simulink library "ENV_Library"  (R2018b)
settings: Solver=VariableStepAuto  StartTime=0.0  StopTime=10.0  RelTol=1e-3
undefined symbols (not defined in the file): c_dif, c_spe, CD, EOP, GM_EARTH, Keddy, leap, mag_data, mass, N_faces, NS, paras_dipole, R_faces, RADIUS_EARTH, RADIUS_SUN, rho_h, S_faces
libraries: MATH_library x7
settings Model: Creator=Andrea  LastModifiedBy=michele

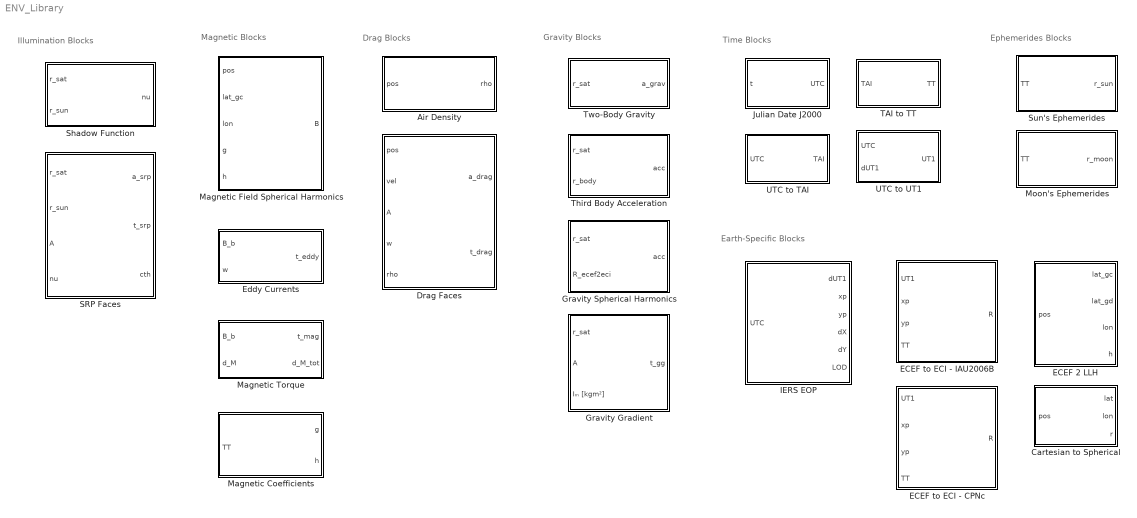
== system ENV_Library ==
  note: Illumination Blocks
  note: Magnetic Blocks
  note: Drag Blocks
  note: Gravity Blocks
  note: Earth-Specific Blocks
  note: Ephemerides Blocks
  note: Time Blocks
  Air Density : Subsystem  mask(Air Density){RBODY=RADIUS_EARTH, rho_h=rho_h}
      mask prompts: RBODY "Body Radius [m]:"; rho_h "Height-Density Look-up Table [km, kg/m³]:"
      mask help: Compute the air density at the input position, given the central body radius and a density look-up table. The input position vector must be expressed in meters.
  Cartesian to Spherical : Subsystem  mask(Cartesian to Spherical){}
      mask help: Transform a position vector in cartesian coordinates into spherical coordinates (geocentric latitude, longitude and radius)
  Drag Faces : Subsystem  mask(Drag Perturbation - Plate Model){CD=CD, m=mass, NS=NS, S_faces=S_faces, N_faces=N_faces, R_faces=R_faces}
      mask prompts: CD "Drag Coefficient [-]:"; m "Spacecraft Mass [kg]:"; NS "Number of Faces"; S_faces "Faces Areas [m²]:"; N_faces "Faces Normals:"; R_faces "Faces Centers wrt CoM [m]:"
      mask help: Compute the drag acceleration and torque by modelling the spacecraft as a collection of plates. It is valid only for the Earth (because it exploits its angular velocity). All the input vectors must be expressed in the Inertial Frame in [m] and [m/s]
      mask DialogControl ParameterGroupVar Prompt: Spacecraft Properties
      mask DialogControl Container3 Prompt: Spacecraft Geometry
  "ECEF 2 LLH  " : Subsystem  mask(ECEF to LLH){}
      mask help: Transform a position vector in ECEF coordinates to geodetic latitude, longitude and altitude from the reference WGS84 ellipsoid. The input vector and output height are expressed in meters.
  ECEF to ECI - CPNc : Subsystem  mask(ECEF to ECI	 - CPNc){}
      mask help:
      | Compute the Position Rotation Matrix from the ECEF to the ECI reference frame using the IERS 2010 Conventions (CPNc approximate Capitaine model) and the Earth Orientation Parameters.
      |
      | The CPNc version is a concise model with a cut-off at 2.5 mas of the X and Y series, delivering a worst-case accuracy of about 15 mas between 1995-2050. It does not take into account the Free Core Nutation (~0.2 mas)
  ECEF to ECI - IAU2006B : Subsystem  mask(ECEF to ECI){}
      mask help: Compute the Position Rotation Matrix from the ECEF to the ECI reference frame using the IERS 2010 Conventions (IAU2006/2000B precession-nutation model) and the Earth Orientation Parameters.
  Eddy Currents : Subsystem  mask(Eddy Currents Torque){Ke=Keddy}
      mask prompts: Ke "Eddy current coefficient:"
      mask help: Compute the magnetic torque induced by Eddy currents in [Nm].
  Gravity Gradient : Subsystem  mask(Gravity Gradient Torque){GM=GM_EARTH}
      mask prompts: GM "Gravitational planetary constant:"
      mask help: Compute the gravity gradient torque in [Nm], given the satellite position, the DCM from the inertial to body frame and the spacecraft inertia matrix. The position vector and the planetary gravitational constant must be expressed in the same units (i.e., m and m³/s²).
  Gravity Spherical Harmonics : Subsystem  mask{GRAV=0}
      mask prompts: GRAV "Spherical Gravity Model Structure:"
      mask DialogControl DescGroupVar Prompt: Gravity Spherical Harmonics
      mask DialogControl DescTextVar Prompt: Compute the perturbing gravitational acceleration using a spherical harmonic expansions. The input position and output acceleration vectors are expressed in the inertial reference frame.
  IERS EOP : Subsystem  mask(Earth Orientation Parameters){EOP=EOP}
      mask prompts: EOP "EOP Data Structure:"
      mask help: Interpolate the IERS EOP data at the given input UTC seconds since J2000.
      mask DialogControl Container2 Prompt: Parameters
  Julian Date J2000 : Subsystem  mask(Julian Date){jd0=0}
      mask prompts: jd0 "Start Julian Date [days]"
      mask help: Return the current simulation time in UTC seconds since J2000. The input time t expresses the seconds elapsed since the starting Julian Date jd0.
  Magnetic Coefficients : Subsystem  mask(Magnetic Field Coefficients){mag_data=0}
      mask prompts: mag_data "Magnetic Field Data:"
      mask help: Compute the magnetic field expansion coefficients at epoch using IGRF's coefficients and their secular variation.
  "Magnetic Field Spherical Harmonics  " : Subsystem  mask(Magnetic Field Vector){mag_data=mag_data}
      mask prompts: mag_data "Magnetic Field Data:"
      mask help: Compute the magnetic field vector in the Inertial frame using the spherical harmonic expansion and IGRF13's coefficients (at epoch). The inputs must be in [m] and [rad].
  Magnetic Torque : Subsystem  mask(Magnetic Torque){parasitic=paras_dipole}
      mask prompts: parasitic "Parasitic Magnetic Dipole [Am²]:"
      mask help: Compute the magnetic perturbing torque in [Nm] given the magnetic field vector in the body frame and the magnetic control dipole.
  Moon's Ephemerides : Subsystem  mask(Moon's Ephemerides){}
      mask help: Compute the Moon's position using low-precision ephemerides. The output position vector is expressed in a True-of-Date geocentric frame in [km].
  "SRP Faces " : Subsystem  mask(SRP Perturbation - Plate Model){m=mass, c_dif=c_dif, c_spe=c_spe, NS=NS, S_faces=S_faces, N_faces=N_faces, R_faces=R_faces}
      mask prompts: m "Spacecraft Mass [kg]:"; c_dif "Diffuse Coefficient [-]:"; c_spe "Specular Coefficient [-]:"; NS "Number of Faces"; S_faces "Faces Areas [m²]:"; N_faces "Faces Normals:"; R_faces "Faces Center of Pressures wrt CoM [m]:"
      mask help: Compute the Solar Radiation Pressure (SRP) acceleration and torque by modelling the spacecraft as a collection of plates. All the input vectors must be in [m]. The shadow function nu is used to trigger the perturbations.
      mask DialogControl ParameterGroupVar Prompt: Spacecraft Properties
      mask DialogControl Container3 Prompt: Optical Properties
      mask DialogControl Container4 Prompt: Spacecraft Geometry
  "Shadow Function " : Subsystem  mask(Shadow Function){Rsun=RADIUS_SUN, Rbody=RADIUS_EARTH}
      mask prompts: Rsun "Radius of the Sun:"; Rbody "Radius of the Occulting Body"
      mask help: Compute the dimensionless shadow function coefficient (i.e., the luminosity ratio). All the inputs must be expressed in the same units.
  Sun's Ephemerides : Subsystem  mask(Sun's Ephemerides){}
      mask help: Compute the Sun's position using low-precision ephemerides. The output position vector is expressed in a True-of-Date geocentric frame in [km].
  TAI to TT : Subsystem  mask(TAI to TT){}
      mask help: Convert seconds since J2000 from the International Atomic Time (TAI) to the Terrestrial Time (TT) scale.
  Third Body Acceleration : Subsystem  mask(Third-Body Perturbation){GM=-3}
      mask prompts: GM "Third: Body Gravitational Constant"
      mask help: Compute the third-body gravitational perturbation, given the spacecraft and the third-body positions with respect to the central body. The input vectors and the planetary gravitational constant must be expressed in the same units of length (i.e., m and m³/s²).
  Two-Body Gravity : Subsystem  mask(Two-Body Acceleration){GM=0}
      mask prompts: GM "Planetary Gravitational Constant:"
      mask help: Compute the gravitational acceleration using the Two-Body Keplerian model. The input vector and the gravitational constant must have the same units of length (i.e., m and m³/s²).
  UTC to TAI : Subsystem  mask(UTC to TAI){leapseconds=leap}
      mask prompts: leapseconds "Leapseconds [s]:"
      mask help: Convert UTC seconds since J2000 to seconds in the International Atomic Time (TAI) scale. This block assumes that no leapseconds are added throughout the simulation.
      mask DialogControl Container2 Prompt: Parameters
  UTC to UT1 : Subsystem  mask(UTC to UT1){}
      mask help: Convert seconds since J2000 from the UTC to the UT1 scale. The additional dUT1 input must also be expressed in seconds.

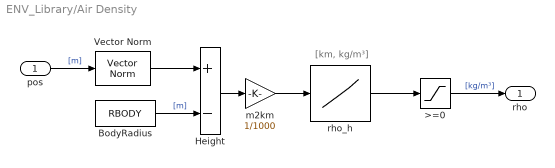
== system ENV_Library/Air Density ==
  note: [km, kg/m³]
  pos : Inport
  >=0 : Saturate  UpperLimit=Inf  LowerLimit=0
  BodyRadius : Constant  Value=RBODY
  Height : Sum  Inputs=+-
  Vector Norm : MATH_library/Vector Norm
  m2km : Gain  Gain=1/1000
  rho_h : Lookup_n-D  NumberOfTableDimensions=1  BreakpointsForDimension1=rho_h(:,1)  Table=rho_h(:,2)  DiagnosticForOutOfRangeInput=Warning  InternalRulePriority=Speed  RndMeth=Simplest  InputSameDT=on
  "rho " : Outport
  wires:
  >=0/1 -> "rho "/1  "[kg/m³]"
  pos/1 -> Vector Norm/1  "[m]"
  rho_h/1 -> >=0/1
  Height/1 -> m2km/1
  BodyRadius/1 -> Height/2  "[m]"
  Vector Norm/1 -> Height/1
  m2km/1 -> rho_h/1

== system ENV_Library/Cartesian to Spherical ==
  note: [m]
  note: [rad]
  note: [m]
  note: [rad]
  pos : Inport
  MATLAB Function : MATLAB Function  TreatAsAtomicUnit=on
  lat : Outport
  lon : Outport  Port=2
  " r" : Outport  Port=3
  wires:
  MATLAB Function/3(r) -> " r"/1
  MATLAB Function/2(lon) -> lon/1
  MATLAB Function/1(lat) -> lat/1
  pos/1 -> MATLAB Function/1(pos)

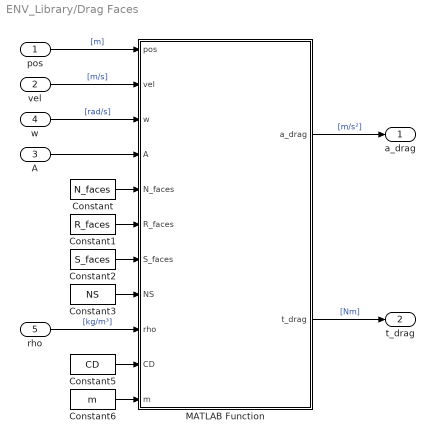
== system ENV_Library/Drag Faces ==
  pos : Inport
  vel : Inport  Port=2
  A : Inport  Port=3
  w : Inport  Port=4
  rho : Inport  Port=5
  Constant : Constant  Value=N_faces
  Constant1 : Constant  Value=R_faces
  Constant2 : Constant  Value=S_faces
  Constant3 : Constant  Value=NS
  Constant5 : Constant  Value=CD
  Constant6 : Constant  Value=m
  MATLAB Function : MATLAB Function  TreatAsAtomicUnit=on
  a_drag : Outport
  t_drag : Outport  Port=2
  wires:
  w/1 -> MATLAB Function/3(w)  "[rad/s]"
  MATLAB Function/2(t_drag) -> t_drag/1  "[Nm]"
  Constant6/1 -> MATLAB Function/11(m)
  Constant5/1 -> MATLAB Function/10(CD)
  rho/1 -> MATLAB Function/9(rho)  "[kg/m³]"
  Constant3/1 -> MATLAB Function/8(NS)
  Constant2/1 -> MATLAB Function/7(S_faces)
  Constant1/1 -> MATLAB Function/6(R_faces)
  Constant/1 -> MATLAB Function/5(N_faces)
  A/1 -> MATLAB Function/4(A)
  MATLAB Function/1(a_drag) -> a_drag/1  "[m/s²]"
  vel/1 -> MATLAB Function/2(vel)  "[m/s]"
  pos/1 -> MATLAB Function/1(pos)  "[m]"

== system ENV_Library/ECEF 2 LLH   ==
  note: [rad]
  note: [m]
  note: [rad]
  note: [m]
  note: [rad]
  pos : Inport
  MATLAB Function : MATLAB Function  TreatAsAtomicUnit=on
  lat_gc : Outport
  lat_gd : Outport  Port=2
  lon : Outport  Port=3
  " h" : Outport  Port=4
  wires:
  MATLAB Function/4(h) -> " h"/1
  MATLAB Function/3(lon) -> lon/1
  MATLAB Function/1(lat_gc) -> lat_gc/1
  pos/1 -> MATLAB Function/1(pos)
  MATLAB Function/2(lat_gd) -> lat_gd/1

== system ENV_Library/ECEF to ECI - CPNc ==
  note: [sec]
  note: [sec]
  note: [rad]
  note: [rad]
  UT1 : Inport
  xp : Inport  Port=2
  yp : Inport  Port=3
  TT : Inport  Port=4
  MATLAB Function : MATLAB Function  TreatAsAtomicUnit=on
  R : Outport
  wires:
  UT1/1 -> MATLAB Function/2(ut1_s)
  MATLAB Function/1(R) -> R/1
  TT/1 -> MATLAB Function/1(tt_s)
  xp/1 -> MATLAB Function/3(xp)
  yp/1 -> MATLAB Function/4(yp)

== system ENV_Library/ECEF to ECI - IAU2006B ==
  UT1 : Inport
  xp : Inport  Port=2
  yp : Inport  Port=3
  TT : Inport  Port=4
  MATLAB Function : MATLAB Function  TreatAsAtomicUnit=on
  R : Outport
  wires:
  yp/1 -> MATLAB Function/4(yp)  "[rad]"
  xp/1 -> MATLAB Function/3(xp)  "[rad]"
  UT1/1 -> MATLAB Function/2(ut1_s)  "[sec]"
  MATLAB Function/1(R) -> R/1
  TT/1 -> MATLAB Function/1(tt_s)  "[sec]"

== system ENV_Library/Eddy Currents ==
  B_b : Inport
  w : Inport  Port=2
  Cross Product : MATH_library/Cross Product
  Cross Product1 : MATH_library/Cross Product
  Gain : Gain  Gain=Ke
  t_eddy : Outport
  wires:
  Gain/1 -> t_eddy/1  "[Nm]"
  Cross Product1/1 -> Gain/1
  B_b/1 -> Cross Product1/2, Cross Product/2  "[T]"
  Cross Product/1 -> Cross Product1/1
  w/1 -> Cross Product/1  "[rad]"

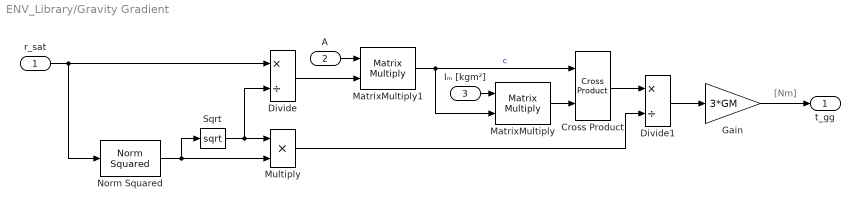
== system ENV_Library/Gravity Gradient ==
  note: [Nm]
  r_sat : Inport
  A : Inport  Port=2
  Iₘ [kgm²] : Inport  Port=3
  Cross Product : MATH_library/Cross Product
  Divide : Product  Inputs=*/
  Divide1 : Product  Inputs=*/
  Gain : Gain  Gain=3*GM
  MatrixMultiply : Product  Multiplication=Matrix(*)
  MatrixMultiply1 : Product  Multiplication=Matrix(*)
  Multiply : Product
  Norm Squared : MATH_library/Norm Squared
  Sqrt : Sqrt  SaturateOnIntegerOverflow=on
  t_gg : Outport
  wires:
  Gain/1 -> t_gg/1
  r_sat/1 -> Norm Squared/1, Divide/1
  Iₘ [kgm²]/1 -> MatrixMultiply/1
  Norm Squared/1 -> Sqrt/1, Multiply/2
  Sqrt/1 -> Divide/2, Multiply/1
  A/1 -> MatrixMultiply1/1
  Divide/1 -> MatrixMultiply1/2
  MatrixMultiply1/1 -> Cross Product/1, MatrixMultiply/2  "c"
  MatrixMultiply/1 -> Cross Product/2
  Cross Product/1 -> Divide1/1
  Multiply/1 -> Divide1/2
  Divide1/1 -> Gain/1

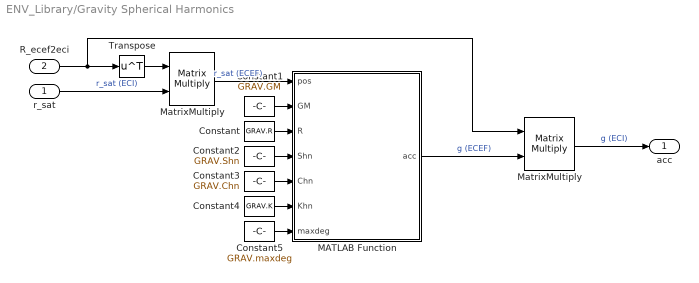
== system ENV_Library/Gravity Spherical Harmonics ==
  r_sat : Inport
  R_ecef2eci : Inport  Port=2
  Constant : Constant  Value=GRAV.R
  Constant1 : Constant  Value=GRAV.GM
  Constant2 : Constant  Value=GRAV.Shn
  Constant3 : Constant  Value=GRAV.Chn
  Constant4 : Constant  Value=GRAV.K
  Constant5 : Constant  Value=GRAV.maxdeg
  MATLAB Function : MATLAB Function  TreatAsAtomicUnit=on
  MatrixMultiply : Product  Multiplication=Matrix(*)
  "MatrixMultiply   " : Product  Multiplication=Matrix(*)
  Transpose : Math  Operator=transpose  SaturateOnIntegerOverflow=on
  acc : Outport
  wires:
  Constant/1 -> MATLAB Function/3(R)
  Constant1/1 -> MATLAB Function/2(GM)
  Constant2/1 -> MATLAB Function/4(Shn)
  Constant3/1 -> MATLAB Function/5(Chn)
  Constant4/1 -> MATLAB Function/6(Khn)
  Constant5/1 -> MATLAB Function/7(maxdeg)
  MatrixMultiply/1 -> acc/1  "g (ECI)"
  MATLAB Function/1(acc) -> MatrixMultiply/2  "g (ECEF)"
  R_ecef2eci/1 -> MatrixMultiply/1, Transpose/1
  "MatrixMultiply   "/1 -> MATLAB Function/1(pos)  "r_sat (ECEF)"
  r_sat/1 -> "MatrixMultiply   "/2  "r_sat (ECI)"
  Transpose/1 -> "MatrixMultiply   "/1

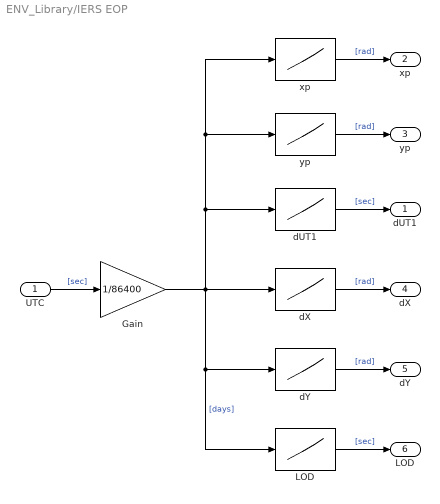
== system ENV_Library/IERS EOP ==
  UTC : Inport
  Gain : Gain  Gain=1/86400
  LOD : Lookup_n-D  NumberOfTableDimensions=1  BreakpointsForDimension1=EOP.jd  Table=EOP.LOD  DiagnosticForOutOfRangeInput=Warning  InternalRulePriority=Speed  RndMeth=Simplest  InputSameDT=on
  dUT1 : Lookup_n-D  NumberOfTableDimensions=1  BreakpointsForDimension1=EOP.jd  Table=EOP.dut1  DiagnosticForOutOfRangeInput=Warning  InternalRulePriority=Speed  RndMeth=Simplest  InputSameDT=on
  dX : Lookup_n-D  NumberOfTableDimensions=1  BreakpointsForDimension1=EOP.jd  Table=EOP.dx  DiagnosticForOutOfRangeInput=Warning  InternalRulePriority=Speed  RndMeth=Simplest  InputSameDT=on
  dY : Lookup_n-D  NumberOfTableDimensions=1  BreakpointsForDimension1=EOP.jd  Table=EOP.dy  DiagnosticForOutOfRangeInput=Warning  InternalRulePriority=Speed  RndMeth=Simplest  InputSameDT=on
  xp : Lookup_n-D  NumberOfTableDimensions=1  BreakpointsForDimension1=EOP.jd  Table=EOP.xp  DiagnosticForOutOfRangeInput=Warning  InternalRulePriority=Speed  RndMeth=Simplest  InputSameDT=on
  yp : Lookup_n-D  NumberOfTableDimensions=1  BreakpointsForDimension1=EOP.jd  Table=EOP.yp  DiagnosticForOutOfRangeInput=Warning  InternalRulePriority=Speed  RndMeth=Simplest  InputSameDT=on
  " dUT1" : Outport
  " xp" : Outport  Port=2
  " yp" : Outport  Port=3
  " dX" : Outport  Port=4
  " dY" : Outport  Port=5
  " LOD" : Outport  Port=6
  wires:
  Gain/1 -> LOD/1, dY/1, dX/1, dUT1/1, yp/1, xp/1  "[days]"
  dY/1 -> " dY"/1  "[rad]"
  LOD/1 -> " LOD"/1  "[sec]"
  dX/1 -> " dX"/1  "[rad]"
  xp/1 -> " xp"/1  "[rad]"
  yp/1 -> " yp"/1  "[rad]"
  UTC/1 -> Gain/1  "[sec]"
  dUT1/1 -> " dUT1"/1  "[sec]"

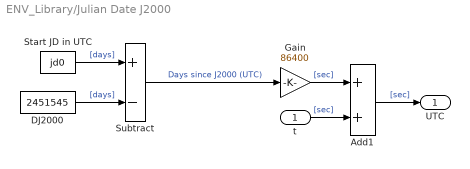
== system ENV_Library/Julian Date J2000 ==
  t : Inport
  Add1 : Sum
  DJ2000 : Constant  Value=2451545
  Gain : Gain  Gain=86400
  "Start JD in UTC " : Constant  Value=jd0
  Subtract : Sum  Inputs=+-
  UTC : Outport
  wires:
  Gain/1 -> Add1/1  "[sec]"
  Subtract/1 -> Gain/1  "Days since J2000 (UTC)"
  DJ2000/1 -> Subtract/2  "[days]"
  "Start JD in UTC "/1 -> Subtract/1  "[days]"
  Add1/1 -> UTC/1  "[sec]"
  t/1 -> Add1/2  "[sec]"

== system ENV_Library/Magnetic Coefficients ==
  note: [sec]
  TT : Inport
  Constant : Constant  Value=mag_data
  MATLAB Function : MATLAB Function  TreatAsAtomicUnit=on
  g : Outport
  h : Outport  Port=2
  wires:
  TT/1 -> MATLAB Function/1(time)
  MATLAB Function/1(g) -> g/1
  MATLAB Function/2(h) -> h/1
  Constant/1 -> MATLAB Function/2(data)

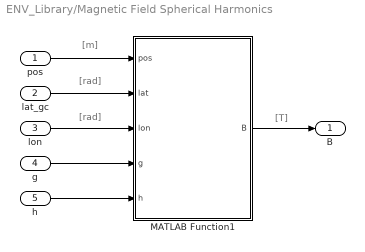
== system ENV_Library/Magnetic Field Spherical Harmonics   ==
  note: [m]
  note: [rad]
  note: [rad]
  note: [T]
  pos : Inport
  lat_gc : Inport  Port=2
  lon : Inport  Port=3
  g : Inport  Port=4
  h : Inport  Port=5
  MATLAB Function1 : MATLAB Function  TreatAsAtomicUnit=on
  B : Outport
  wires:
  g/1 -> MATLAB Function1/4(g)
  pos/1 -> MATLAB Function1/1(pos)
  lon/1 -> MATLAB Function1/3(lon)
  lat_gc/1 -> MATLAB Function1/2(lat)
  MATLAB Function1/1(B) -> B/1
  h/1 -> MATLAB Function1/5(h)

== system ENV_Library/Magnetic Torque ==
  note: [T]
  note: [Am²]
  note: [Nm]
  note: [Am²]
  B_b : Inport
  d_M : Inport  Port=2
  Constant : Constant  Value=parasitic
  Cross Product : MATH_library/Cross Product
  Subtract : Sum
  t_mag : Outport
  d_M_tot : Outport  Port=2
  wires:
  Cross Product/1 -> t_mag/1
  Subtract/1 -> Cross Product/1, d_M_tot/1
  Constant/1 -> Subtract/2
  d_M/1 -> Subtract/1
  B_b/1 -> Cross Product/2

== system ENV_Library/Moon's Ephemerides ==
  TT : Inport
  MoonEphemeris : MATLAB Function  TreatAsAtomicUnit=on
  r_moon : Outport
  wires:
  MoonEphemeris/1(pos) -> r_moon/1
  TT/1 -> MoonEphemeris/1(time)  "[sec]"

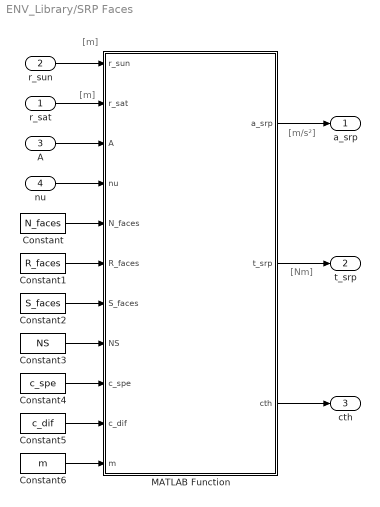
== system ENV_Library/SRP Faces  ==
  note: [m]
  note: [m]
  note: [Nm]
  note: [m/s²]
  r_sat : Inport
  r_sun : Inport  Port=2
  A : Inport  Port=3
  nu : Inport  Port=4
  Constant : Constant  Value=N_faces
  Constant1 : Constant  Value=R_faces
  Constant2 : Constant  Value=S_faces
  Constant3 : Constant  Value=NS
  Constant4 : Constant  Value=c_spe
  Constant5 : Constant  Value=c_dif
  Constant6 : Constant  Value=m
  MATLAB Function : MATLAB Function  TreatAsAtomicUnit=on
  a_srp : Outport
  t_srp : Outport  Port=2
  cth : Outport  Port=3
  wires:
  MATLAB Function/3(cth) -> cth/1
  MATLAB Function/2(t_srp) -> t_srp/1
  Constant6/1 -> MATLAB Function/11(m)
  Constant5/1 -> MATLAB Function/10(c_dif)
  Constant4/1 -> MATLAB Function/9(c_spe)
  Constant3/1 -> MATLAB Function/8(NS)
  Constant2/1 -> MATLAB Function/7(S_faces)
  Constant1/1 -> MATLAB Function/6(R_faces)
  Constant/1 -> MATLAB Function/5(N_faces)
  nu/1 -> MATLAB Function/4(nu)
  A/1 -> MATLAB Function/3(A)
  r_sun/1 -> MATLAB Function/1(r_sun)
  r_sat/1 -> MATLAB Function/2(r_sat)
  MATLAB Function/1(a_srp) -> a_srp/1

== system ENV_Library/Shadow Function  ==
  note: [m]
  note: [m]
  r_sat : Inport
  r_sun : Inport  Port=2
  Constant : Constant  Value=Rsun
  Constant1 : Constant  Value=Rbody
  MATLAB Function : MATLAB Function  TreatAsAtomicUnit=on
  nu : Outport
  wires:
  Constant1/1 -> MATLAB Function/4(Rp)
  Constant/1 -> MATLAB Function/3(Rs)
  r_sun/1 -> MATLAB Function/2(r_sun)
  r_sat/1 -> MATLAB Function/1(r_sat)
  MATLAB Function/1(nu) -> nu/1

== system ENV_Library/Sun's Ephemerides ==
  TT : Inport
  SunEphemeris : MATLAB Function  TreatAsAtomicUnit=on
  r_sun : Outport
  wires:
  SunEphemeris/1(pos) -> r_sun/1
  TT/1 -> SunEphemeris/1(time)  "[sec]"

== system ENV_Library/TAI to TT ==
  TAI : Inport
  Add1 : Sum
  Constant : Constant  Value=32.184
  TT : Outport
  wires:
  Constant/1 -> Add1/1  "[sec]"
  Add1/1 -> TT/1  "[sec]"
  TAI/1 -> Add1/2  "[sec]"

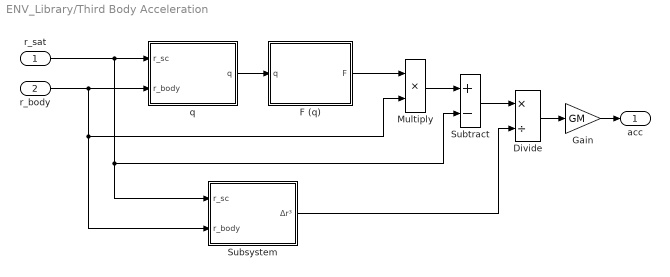
== system ENV_Library/Third Body Acceleration ==
  r_sat : Inport
  r_body : Inport  Port=2
  Divide : Product  Inputs=*/
  F (q) : Subsystem
  Gain : Gain  Gain=GM
  Multiply : Product
  Subsystem : Subsystem
  Subtract : Sum  Inputs=+-
  q : Subsystem
  acc : Outport
  wires:
  r_sat/1 -> Subsystem/1(r_sc), Subtract/2, q/1(r_sc)
  q/1(q) -> F (q)/1(q)
  r_body/1 -> Subsystem/2(r_body), Multiply/2, q/2(r_body)
  F (q)/1(F) -> Multiply/1
  Multiply/1 -> Subtract/1
  Subtract/1 -> Divide/1
  Subsystem/1(Δr³) -> Divide/2
  Divide/1 -> Gain/1
  Gain/1 -> acc/1

== system ENV_Library/Two-Body Gravity ==
  r_sat : Inport
  Divide : Product  Inputs=*/
  Gain : Gain  Gain=-GM
  Multiply : Product
  Norm Squared : MATH_library/Norm Squared
  Sqrt : Sqrt  SaturateOnIntegerOverflow=on
  a_grav : Outport
  wires:
  Gain/1 -> a_grav/1
  Norm Squared/1 -> Multiply/1, Sqrt/1
  r_sat/1 -> Norm Squared/1, Divide/1
  Divide/1 -> Gain/1
  Sqrt/1 -> Multiply/2
  Multiply/1 -> Divide/2

== system ENV_Library/UTC to TAI ==
  UTC : Inport
  Constant : Constant  Value=leapseconds
  Subtract : Sum
  TAI : Outport
  wires:
  Subtract/1 -> TAI/1  "[sec]"
  UTC/1 -> Subtract/2  "[sec]"
  Constant/1 -> Subtract/1  "[sec]"

== system ENV_Library/UTC to UT1 ==
  UTC : Inport
  dUT1 : Inport  Port=2
  Add1 : Sum
  UT1 : Outport
  wires:
  dUT1/1 -> Add1/1  "[sec]"
  Add1/1 -> UT1/1  "[sec]"
  UTC/1 -> Add1/2  "[sec]"

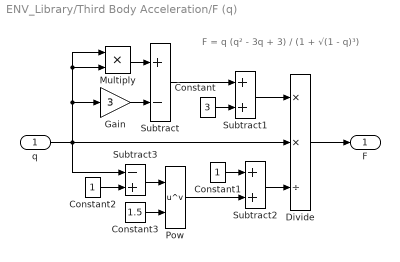
== system ENV_Library/Third Body Acceleration/F (q) ==
  note: F = q (q² - 3q + 3) / (1 + √(1 - q)³)
  q : Inport
  Constant : Constant  Value=3
  Constant1 : Constant
  Constant2 : Constant
  Constant3 : Constant  Value=1.5
  Divide : Product  Inputs=**/
  Gain : Gain  Gain=3
  Multiply : Product
  Pow : Math  Operator=pow  RndMeth=Zero  SaturateOnIntegerOverflow=on
  Subtract : Sum  Inputs=+-
  Subtract1 : Sum
  Subtract2 : Sum
  Subtract3 : Sum  Inputs=-+
  F : Outport
  wires:
  q/1 -> Divide/2, Subtract3/1, Gain/1, Multiply/2, Multiply/1
  Multiply/1 -> Subtract/1
  Gain/1 -> Subtract/2
  Subtract/1 -> Subtract1/1
  Constant/1 -> Subtract1/2
  Subtract1/1 -> Divide/1
  Divide/1 -> F/1
  Subtract2/1 -> Divide/3
  Subtract3/1 -> Pow/1
  Constant3/1 -> Pow/2
  Constant1/1 -> Subtract2/1
  Pow/1 -> Subtract2/2
  Constant2/1 -> Subtract3/2

== system ENV_Library/Third Body Acceleration/Subsystem ==
  r_sc : Inport
  r_body : Inport  Port=2
  Dot Product : DotProduct  InputSameDT=on  OutDataTypeStr=Inherit: Inherit via internal rule
  Multiply : Product
  Sqrt : Sqrt  SaturateOnIntegerOverflow=on
  Subtract : Sum  Inputs=+-
  Δr³ : Outport
  wires:
  r_sc/1 -> Subtract/1
  r_body/1 -> Subtract/2
  Multiply/1 -> Δr³/1
  Subtract/1 -> Dot Product/1, Dot Product/2
  Sqrt/1 -> Multiply/2
  Dot Product/1 -> Multiply/1, Sqrt/1

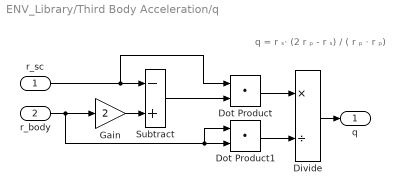
== system ENV_Library/Third Body Acceleration/q ==
  note: q = r ₛ⋅ (2 r ₚ - r ₛ) / ( r ₚ ⋅ r ₚ)
  r_sc : Inport
  r_body : Inport  Port=2
  Divide : Product  Inputs=*/
  Dot Product : DotProduct  InputSameDT=on  OutDataTypeStr=Inherit: Inherit via internal rule
  Dot Product1 : DotProduct  InputSameDT=on  OutDataTypeStr=Inherit: Inherit via internal rule
  Gain : Gain  Gain=2
  Subtract : Sum  Inputs=-+
  q : Outport
  wires:
  Gain/1 -> Subtract/2
  r_sc/1 -> Dot Product/1, Subtract/1
  r_body/1 -> Dot Product1/1, Dot Product1/2, Gain/1
  Subtract/1 -> Dot Product/2
  Dot Product/1 -> Divide/1
  Dot Product1/1 -> Divide/2
  Divide/1 -> q/1

== matlab function ENV_Library/ECEF to ECI - CPNc/MATLAB Function ==
  data: R output; tt_s input; ut1_s input; xp input; yp input
function R = ecef2eci(tt_s, ut1_s, xp, yp)
   
    % Convert a position vector from ECI to ECEF coordinates using 
    % following the IAU2010 conventions and IERS EOP parameters.
    R = rot3_ecef2eci_cpnc(tt_s, ut1_s, xp, yp);
    
end

== matlab function ENV_Library/Sun's Ephemerides/SunEphemeris ==
  data: time input; pos output
function pos = sun(time)
    
    % Compute the geocentric position of the Sun in the ECI frame (km)
    [~, ~, pos] = ephem_sun(time);

end

== matlab function ENV_Library/Magnetic Coefficients/MATLAB Function ==
  data: time input; g output; data input; h output
function [g, h] = get_coeffs(time, data)

    % Compute IGRF13's coefficients at epoch
    [g, h] = get_magnetic_coeffs(time, data);

end

== matlab function ENV_Library/Moon's Ephemerides/MoonEphemeris ==
  data: time input; pos output
function pos = moon(time)
    
    % Compute the geocentric position of the Moon in the ECI frame (km)
    [~, ~, pos] = ephem_moon(time);

end

== matlab function ENV_Library/Gravity Spherical Harmonics/MATLAB Function ==
  data: pos input; GM input; acc output; R input; Shn input; Chn input; Khn input; maxdeg input
function acc = gravity_acc(pos, GM, R, Shn, Chn, Khn, maxdeg)
    
    % Compute the perturbing gravitational acceleration in body-fixed 
    % coordinates using the spherical harmonic expansion. See
    % gravity_field_spherical.m documentation for more insights. 
    
    acc = gravity_field_spherical(pos, GM, R, Shn, Chn, Khn, maxdeg);

end

== matlab function ENV_Library/ECEF to ECI - IAU2006B/MATLAB Function ==
  data: R output; tt_s input; ut1_s input; xp input; yp input
function R = ecef2eci(tt_s, ut1_s, xp, yp)
   
    % Convert a position vector from ECI to ECEF coordinates using 
    % following the IAU2010 conventions and IERS EOP parameters.
    R = rot3_ecef2eci_iau2006b(tt_s, ut1_s, xp, yp);
    
end

== matlab function ENV_Library/Drag Faces/MATLAB Function ==
  data: pos input; a_drag output; vel input; w input; A input; N_faces input; R_faces input; S_faces input; NS input; rho input; CD input; m input; t_drag output
function [a_drag, t_drag] = drag_face(pos, vel, w, A, N_faces, R_faces, ...
                                    S_faces, NS, rho, CD, m)
                                
    % Compute the Drag acceleration and Torque by modelling the spacecraft 
    % as a collection of plates.
    
    % See drag_faces.m documentation for more insights.
    
    [a_drag, t_drag] = drag_faces(pos, vel, w, A, rho, N_faces, R_faces, ... 
                                S_faces, NS, CD, m);
    

end

== matlab function ENV_Library/Magnetic Field Spherical Harmonics  /MATLAB Function1 ==
  data: pos input; B output; lat input; lon input; g input; h input
function B = mag_field(pos, lat, lon, g, h)
    
    % Compute the magnetic field vector in the inertial frame. 
    % Check magnetic_field_spherical.m documentation for more info.

    B = magnetic_field_spherical(pos, lat, lon, g, h);

end

== matlab function ENV_Library/ECEF 2 LLH  /MATLAB Function ==
  data: pos input; lat_gc output; lat_gd output; lon output; h output
function [lat_gc, lat_gd, lon, h] = to_llh(pos)

    % Transform a position vector in the ECEF frame into geodetic
    % longitude, latitude and altitude over the WGS-84 ellipsoid. 
    % Check ecef2llh.m documentation for more information.

    [lat_gd, lon, h] = ecef2llh(pos);
    [lat_gc, ~, ~] = pos2geoc(pos);

    
end

== matlab function ENV_Library/Cartesian to Spherical/MATLAB Function ==
  data: pos input; lat output; lon output; r output
function [lat, lon, r] = pos_to_geoc(pos)


    [lat, lon, r] = pos2geoc(pos);

    
end

== matlab function ENV_Library/Shadow Function /MATLAB Function ==
  data: r_sat input; nu output; r_sun input; Rs input; Rp input
function nu = illumination(r_sat, r_sun, Rs, Rp)

    % Compute the shadow function from a generic occulting body. 
    % See shadow_function.m documentation for more info.
    
    nu = shadow_function(r_sat, r_sun, Rs, Rp);
    
end

== matlab function ENV_Library/SRP Faces /MATLAB Function ==
  data: r_sun input; a_srp output; r_sat input; A input; nu input; N_faces input; R_faces input; S_faces input; NS input; c_spe input; c_dif input; m input; t_srp output; cth output
function [a_srp, t_srp, cth] = srp_face(r_sun, r_sat, A, nu, N_faces, R_faces, ...
                                    S_faces, NS, c_spe, c_dif, m)
                                
    % Compute the Solar Radiation Pressure (SRP) acceleration and Torque 
    % by modelling the spacecraft as a collection of plates.
    
    % See srp_faces.m documentation for more insights.
    
    [a_srp, t_srp, cth] = srp_faces(r_sun, r_sat, A, nu, N_faces, R_faces, ...
                            S_faces, NS, c_spe, c_dif, m);
    

end
